simulink model "robust_controller"  (Simulink 7.2)
settings: Solver=FixedStepDiscrete  SolverMode=SingleTasking  StartTime=0  StopTime=inf  FixedStep=TS  RelTol=1e-3
PreLoadFcn:
  | param_nxtway_gs
values from neighbouring files (symbols this model uses):
  C_hh = [1 0]    [olp_robot_2dof.m]
undefined symbols (not defined in the file or in its folder): a_b, a_d, a_gc, a_gd, A_h, a_r, B_h, C_h, D_h, dst_thr, gp_max, k_phidot, k_sync, k_thetadot, log_count, pwm_gain, sound_dur, sound_freq, time_auto, time_start, ts1, ts2, ts3, turn_angle
libraries: ecrobot_nxt_lib x30, simulink x2
(part 1 of 2)
settings Model: Creator=y_yama  LastModifiedBy=Petko Petkov
settings DataIOCC: SaveOutput=off  SignalLogging=off  SaveTime=off
settings OptimizationCC: InlineParams=on  InlineInvariantSignals=on  EnforceIntegerDowncast=off  RollThreshold=2  StateBitsets=on  DataBitsets=on  UseTempVars=on  ZeroExternalMemoryAtStartup=off  ZeroInternalMemoryAtStartup=off  InitFltsAndDblsToZero=on  NoFixptDivByZeroProtection=on  EfficientFloat2IntCast=on  OptimizeModelRefInitCode=on  LifeSpan=1
settings DebuggingCC: ConsistencyChecking=warning  SignalInfNanChecking=warning  ReadBeforeWriteMsg=DisableAll  WriteAfterWriteMsg=DisableAll  WriteAfterReadMsg=DisableAll  AlgebraicLoopMsg=error  CheckExecutionContextPreStartOutputMsg=on  CheckExecutionContextRuntimeOutputMsg=on  SolverPrmCheckMsg=none  MultiTaskDSMMsg=warning  SingleTaskRateTransMsg=warning  TasksWithSamePriorityMsg=none  IntegerOverflowMsg=none  ParameterPrecisionLossMsg=none  UnconnectedInputMsg=error  UnconnectedOutputMsg=error  UnconnectedLineMsg=error  UniqueDataStoreMsg=error  BusObjectLabelMismatch=error  RootOutportRequireBusObject=error
settings HardwareCC: ProdIntDivRoundTo=Zero  ProdEndianess=LittleEndian  ProdHWDeviceType=ARM7  TargetHWDeviceType=32-bit Generic
settings ModelReferenceCC: ModelReferenceNumInstancesAllowed=Single
settings RTWCC: SystemTargetFile=ert.tlc  GenCodeOnly=on  GenerateMakefile=off  TemplateMakefile=ert_default_tmf  Description=Real-Time Workshop Embedded Coder (no auto configuration)  GenerateReport=on  RTWVerbose=off  ProcessScript=ert_make_rtw_hook  IncludeHyperlinkInReport=on  LaunchReport=on
settings CodeAppCC: ForceParamTrailComments=on  IgnoreCustomStorageClasses=off  MaxIdLength=63  SFDataObjDesc=on  CustomSymbolStrGlobalVar=rt$N$M  CustomSymbolStrType=$N$M  CustomSymbolStrFcn=$N$M$F  CustomSymbolStrMacro=$N$M  InsertBlockDesc=on
settings ERTTargetCC: TargetFcnLib=ansi_tfl_tmw.mat  TargetFunctionLibrary=GNU  MultiwordLength=2048  IncludeMdlTerminateFcn=off  SuppressErrorStatus=on  SupportAbsoluteTime=off  SupportNonFinite=off  SupportComplex=off  InlinedParameterPlacement=NonHierarchical  RootIOFormat=Structure reference  ERTCustomFileTemplate=example_file_process.tlc

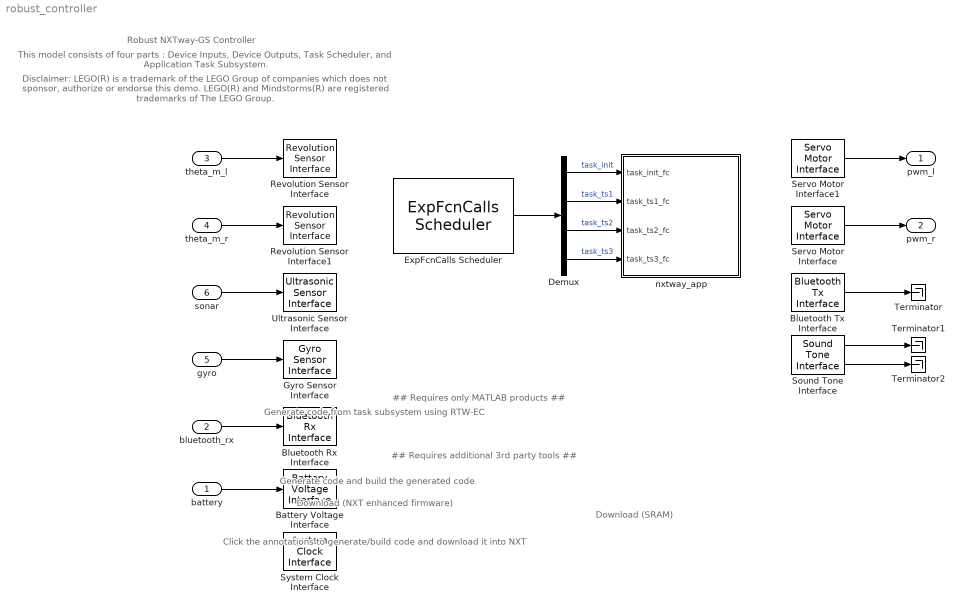
== system robust_controller ==
  note: Disclaimer:
      | LEGO(R) is a trademark of the LEGO Group of companies which does not sponsor, authorize or endorse this demo.
      | LEGO(R) and Mindstorms(R) are registered trademarks of The LEGO Group.
  note: Robust NXTway-GS Controller
  note: This model consists of four parts : Device Inputs, Device Outputs, Task Scheduler, and Application Task Subsystem.
  note: Generate code from task subsystem using RTW-EC
  note: Generate code and build the generated code
  note: ## Requires only MATLAB products ##
  note: ## Requires additional 3rd party tools ##
  note: Download (SRAM)
  note: Download (NXT enhanced firmware)
  note: Click the annotations to generate/build code and download it into NXT
  battery : Inport  DataType=uint16  OutDataType=sfix(16)  OutScaling=2^0  OutDataTypeStr=uint16
  bluetooth_rx : Inport  Port=2  DataType=uint8  OutDataType=sfix(16)  OutScaling=2^0  OutDataTypeStr=uint8
  theta_m_l : Inport  Port=3  DataType=int32  OutDataType=sfix(16)  OutScaling=2^0  OutDataTypeStr=int32
  theta_m_r : Inport  Port=4  DataType=int32  OutDataType=sfix(16)  OutScaling=2^0  OutDataTypeStr=int32
  gyro : Inport  Port=5  DataType=uint16  OutDataType=sfix(16)  OutScaling=2^0  OutDataTypeStr=uint16
  sonar : Inport  Port=6  DataType=int32  OutDataType=sfix(16)  OutScaling=2^0  OutDataTypeStr=int32
  Battery Voltage Interface : ecrobot_nxt_lib/Battery Voltage Interface  Priority=-1  SystemSampleTime=-1
      settings: AttributesFormatString=Priority = %<Priority>
  Bluetooth Rx Interface : ecrobot_nxt_lib/Bluetooth Rx Interface  Priority=-1  SystemSampleTime=-1
      settings: AttributesFormatString=Priority = %<Priority>
  Bluetooth Tx Interface : ecrobot_nxt_lib/Bluetooth Tx Interface  Priority=1  SystemSampleTime=-1
      settings: AttributesFormatString=Priority = %<Priority>
  Demux : Demux
  ExpFcnCalls Scheduler : ecrobot_nxt_lib/ExpFcnCalls Scheduler  Priority=0  fcname='task_init', 'task_ts1', 'task_ts2', 'task_ts3'  fctrigger=[0, ts1*1000, ts2*1000, ts3*1000]  ts=0.001  platform=OSEK  stacksize=[512, 512, 512, 512]  bd_mode=Slave
      settings: AttributesFormatString=Priority = %<Priority>
  Gyro Sensor Interface : ecrobot_nxt_lib/Gyro Sensor Interface  Priority=-1  SystemSampleTime=-1  ip=S4
      settings: AttributesFormatString=Port = %<ip>\nPriority = %<Priority>
  Revolution Sensor Interface : ecrobot_nxt_lib/Revolution Sensor Interface  Priority=-1  SystemSampleTime=-1  ip=C
      settings: AttributesFormatString=Port = %<ip>\nPriority = %<Priority>
  Revolution Sensor Interface1 : ecrobot_nxt_lib/Revolution Sensor Interface  Priority=-1  SystemSampleTime=-1  ip=B
      settings: AttributesFormatString=Port = %<ip>\nPriority = %<Priority>
  Servo Motor Interface : ecrobot_nxt_lib/Servo Motor Interface  Priority=1  SystemSampleTime=-1  ip=B  mode=Brake
      settings: AttributesFormatString=Port = %<ip>\nPriority = %<Priority>
  Servo Motor Interface1 : ecrobot_nxt_lib/Servo Motor Interface  Priority=1  SystemSampleTime=-1  ip=C  mode=Brake
      settings: AttributesFormatString=Port = %<ip>\nPriority = %<Priority>
  Sound Tone Interface : ecrobot_nxt_lib/Sound Tone  Interface  Priority=1  SystemSampleTime=-1
      settings: AttributesFormatString=Priority = %<Priority>
  System Clock Interface : ecrobot_nxt_lib/System Clock Interface  Priority=-1  SystemSampleTime=-1
      settings: AttributesFormatString=Priority = %<Priority>
  Terminator : Terminator
  Terminator1 : Terminator
  Terminator2 : Terminator
  Ultrasonic Sensor Interface : ecrobot_nxt_lib/Ultrasonic Sensor Interface  Priority=-1  SystemSampleTime=-1  ip=S2
      settings: AttributesFormatString=Port = %<ip>\nPriority = %<Priority>
  nxtway_app : Subsystem
  pwm_l : Outport  OutDataType=sfix(16)  OutScaling=2^0
  pwm_r : Outport  Port=2  OutDataType=sfix(16)  OutScaling=2^0
  wires:
  sonar/1 -> Ultrasonic Sensor Interface/1
  gyro/1 -> Gyro Sensor Interface/1
  theta_m_r/1 -> Revolution Sensor Interface1/1
  theta_m_l/1 -> Revolution Sensor Interface/1
  ExpFcnCalls Scheduler/1 -> Demux/1
  Bluetooth Tx Interface/1 -> Terminator/1
  Servo Motor Interface/1 -> pwm_r/1
  Servo Motor Interface1/1 -> pwm_l/1
  bluetooth_rx/1 -> Bluetooth Rx Interface/1
  battery/1 -> Battery Voltage Interface/1
  Demux/1 -> nxtway_app/1(task_init_fc)  "task_init"
  Demux/2 -> nxtway_app/2(task_ts1_fc)  "task_ts1"
  Demux/3 -> nxtway_app/3(task_ts2_fc)  "task_ts2"
  Demux/4 -> nxtway_app/4(task_ts3_fc)  "task_ts3"
  Sound Tone Interface/1 -> Terminator1/1
  Sound Tone Interface/2 -> Terminator2/1

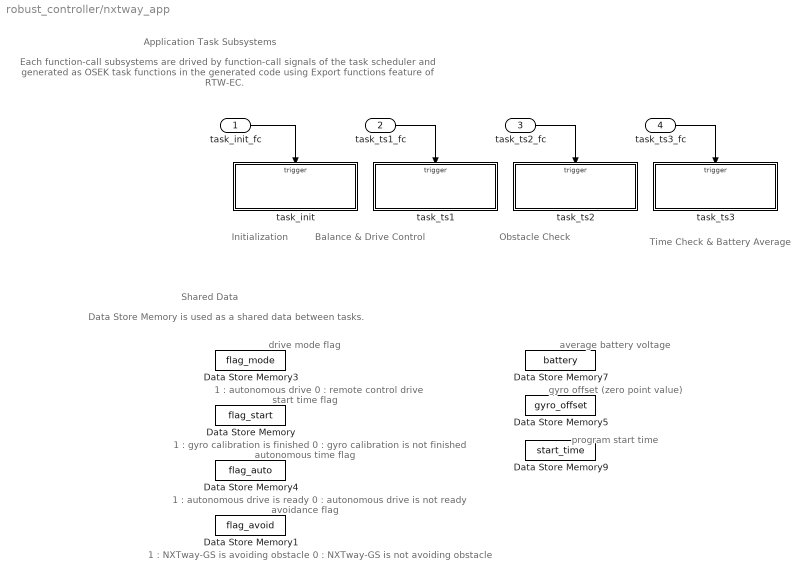
== system robust_controller/nxtway_app ==
  note: Application Task Subsystems
  note: Each function-call subsystems are drived by function-call signals of the task scheduler and
      | generated as OSEK task functions in the generated code using Export functions feature of RTW-EC.
  note: Initialization
  note: Balance & Drive Control
  note: Time Check &
      | Battery Average
  note: Shared Data
  note: Data Store Memory is used as a shared data between tasks.
  note: drive mode flag
  note: 1 : autonomous drive
      | 0 : remote control drive
  note: start time flag
  note: 1 : gyro calibration is finished
      | 0 : gyro calibration is not finished
  note: autonomous time flag
  note: 1 : autonomous drive is ready
      | 0 : autonomous drive is not ready
  note: average battery voltage
  note: gyro offset (zero point value)
  note: program start time
  note: Obstacle Check
  note: avoidance flag
  note: 1 : NXTway-GS is avoiding obstacle
      | 0 : NXTway-GS is not avoiding obstacle
  task_init_fc : Inport  OutDataType=sfix(16)  OutScaling=2^0
  task_ts1_fc : Inport  Port=2  OutDataType=sfix(16)  OutScaling=2^0
  task_ts2_fc : Inport  Port=3  OutDataType=sfix(16)  OutScaling=2^0
  task_ts3_fc : Inport  Port=4  OutDataType=sfix(16)  OutScaling=2^0
  Data Store Memory : DataStoreMemory  DataStoreName=flag_start  ReadBeforeWriteMsg=warning  WriteAfterWriteMsg=warning  WriteAfterReadMsg=warning  DataType=boolean  OutDataType=sfix(16)  OutScaling=2^0  OutDataTypeStr=boolean
      settings: AttributesFormatString=DataType = %<OutDataTypeStr>
  Data Store Memory1 : DataStoreMemory  DataStoreName=flag_avoid  ReadBeforeWriteMsg=warning  WriteAfterWriteMsg=warning  WriteAfterReadMsg=warning  DataType=boolean  OutDataType=sfix(16)  OutScaling=2^0  OutDataTypeStr=boolean
      settings: AttributesFormatString=DataType = %<OutDataTypeStr>
  Data Store Memory3 : DataStoreMemory  DataStoreName=flag_mode  ReadBeforeWriteMsg=warning  WriteAfterWriteMsg=warning  WriteAfterReadMsg=warning  DataType=boolean  OutDataType=sfix(16)  OutScaling=2^0  OutDataTypeStr=boolean
      settings: AttributesFormatString=DataType = %<OutDataTypeStr>
  Data Store Memory4 : DataStoreMemory  DataStoreName=flag_auto  ReadBeforeWriteMsg=warning  WriteAfterWriteMsg=warning  WriteAfterReadMsg=warning  DataType=boolean  OutDataType=sfix(16)  OutScaling=2^0  OutDataTypeStr=boolean
      settings: AttributesFormatString=DataType = %<OutDataTypeStr>
  Data Store Memory5 : DataStoreMemory  DataStoreName=gyro_offset  ReadBeforeWriteMsg=warning  WriteAfterWriteMsg=warning  WriteAfterReadMsg=warning  DataType=single  OutDataType=sfix(16)  OutScaling=2^0  OutDataTypeStr=single
      settings: AttributesFormatString=DataType = %<OutDataTypeStr>
  Data Store Memory7 : DataStoreMemory  DataStoreName=battery  ReadBeforeWriteMsg=warning  WriteAfterWriteMsg=warning  WriteAfterReadMsg=warning  DataType=single  OutDataType=sfix(16)  OutScaling=2^0  OutDataTypeStr=single
      settings: AttributesFormatString=DataType = %<OutDataTypeStr>
  Data Store Memory9 : DataStoreMemory  DataStoreName=start_time  ReadBeforeWriteMsg=warning  WriteAfterWriteMsg=warning  WriteAfterReadMsg=warning  DataType=uint32  OutDataType=sfix(16)  OutScaling=2^0  OutDataTypeStr=uint32
      settings: AttributesFormatString=DataType = %<OutDataTypeStr>
  task_init : Subsystem  TreatAsAtomicUnit=on
  task_ts1 : Subsystem  TreatAsAtomicUnit=on
  task_ts2 : Subsystem  TreatAsAtomicUnit=on
  task_ts3 : Subsystem  TreatAsAtomicUnit=on
  wires:
  task_init_fc/1 -> task_init/Trigger
  task_ts1_fc/1 -> task_ts1/Trigger
  task_ts3_fc/1 -> task_ts3/Trigger
  task_ts2_fc/1 -> task_ts2/Trigger

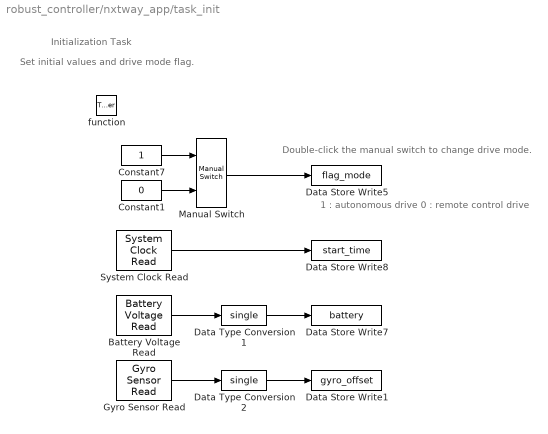
== system robust_controller/nxtway_app/task_init ==
  note: Initialization Task
  note: Set initial values and drive mode flag.
  note: Double-click the manual switch
      |  to change drive mode.
  note: 1 : autonomous drive
      | 0 : remote control drive
  function : TriggerPort  TriggerType=function-call
  Battery Voltage Read : ecrobot_nxt_lib/Battery Voltage Read  SystemSampleTime=-1
  Constant1 : Constant  Value=0  OutDataTypeMode=boolean  OutDataType=sfix(16)  OutScaling=2^0  OutDataTypeStr=boolean  SampleTime=-1
      settings: AttributesFormatString=DataType = %<OutDataTypeStr>
  Constant7 : Constant  OutDataTypeMode=boolean  OutDataType=sfix(16)  OutScaling=2^0  OutDataTypeStr=boolean  SampleTime=-1
      settings: AttributesFormatString=DataType = %<OutDataTypeStr>
  Data Store Write1 : DataStoreWrite  DataStoreName=gyro_offset  SampleTime=-1
  Data Store Write5 : DataStoreWrite  DataStoreName=flag_mode  SampleTime=-1
  Data Store Write7 : DataStoreWrite  DataStoreName=battery  SampleTime=-1
  Data Store Write8 : DataStoreWrite  DataStoreName=start_time  SampleTime=-1
  Data Type Conversion1 : DataTypeConversion  OutDataTypeMode=single  OutDataType=sfix(16)  OutScaling=2^0  OutDataTypeStr=single  RndMeth=Simplest
      settings: AttributesFormatString=Round = %<RndMeth>
  Data Type Conversion2 : DataTypeConversion  OutDataTypeMode=single  OutDataType=sfix(16)  OutScaling=2^0  OutDataTypeStr=single  RndMeth=Simplest
      settings: AttributesFormatString=Round = %<RndMeth>
  Gyro Sensor Read : ecrobot_nxt_lib/Gyro Sensor Read  SystemSampleTime=-1  ip=S4
      settings: AttributesFormatString=Port = %<ip>
  Manual Switch : simulink/Signal Routing/Manual Switch  SystemSampleTime=-1  sw=0  action=0  varsize=off
  System Clock Read : ecrobot_nxt_lib/System Clock Read  SystemSampleTime=-1
  wires:
  Gyro Sensor Read/1 -> Data Type Conversion2/1
  Data Type Conversion2/1 -> Data Store Write1/1
  Battery Voltage Read/1 -> Data Type Conversion1/1
  Data Type Conversion1/1 -> Data Store Write7/1
  Constant7/1 -> Manual Switch/1
  Constant1/1 -> Manual Switch/2
  Manual Switch/1 -> Data Store Write5/1
  System Clock Read/1 -> Data Store Write8/1

== system robust_controller/nxtway_app/task_ts1 ==
  note: Balance & Drive Control Task
  note: Control NXTway-GS to balance itself and drive autonomously or
      | by remote control after gyro calibration.
  function : TriggerPort  TriggerType=function-call
  Balance & Drive Control : Subsystem
  Data Store Read : DataStoreRead  DataStoreName=flag_start  SampleTime=-1
  Gyro Calibration : Subsystem  TreatAsAtomicUnit=on
  Logical Operator : Logic  Operator=NOT  AllPortsSameDT=off  OutDataTypeMode=boolean  OutDataTypeStr=boolean
  wires:
  Data Store Read/1 -> Logical Operator/1, Balance & Drive Control/Enable
  Logical Operator/1 -> Gyro Calibration/Enable

== system robust_controller/nxtway_app/task_ts2 ==
  note: Get the distance between NXTway-GS and obstacle using the ultrasonic sensor.
      | NXTway-GS rotates right in autonomous drive mode and runs backward in remote
      | control drive mode when the distance is under the threshold.
  note: Obstacle Check Task
  function : TriggerPort  TriggerType=function-call
  Autonomous Drive : Subsystem
  Data Store Read1 : DataStoreRead  DataStoreName=flag_mode  SampleTime=-1
  Logical Operator : Logic  Operator=NOT  AllPortsSameDT=off  OutDataTypeMode=boolean  OutDataTypeStr=boolean
  Remote Control Drive : Subsystem
  wires:
  Logical Operator/1 -> Remote Control Drive/Enable
  Data Store Read1/1 -> Logical Operator/1, Autonomous Drive/Enable

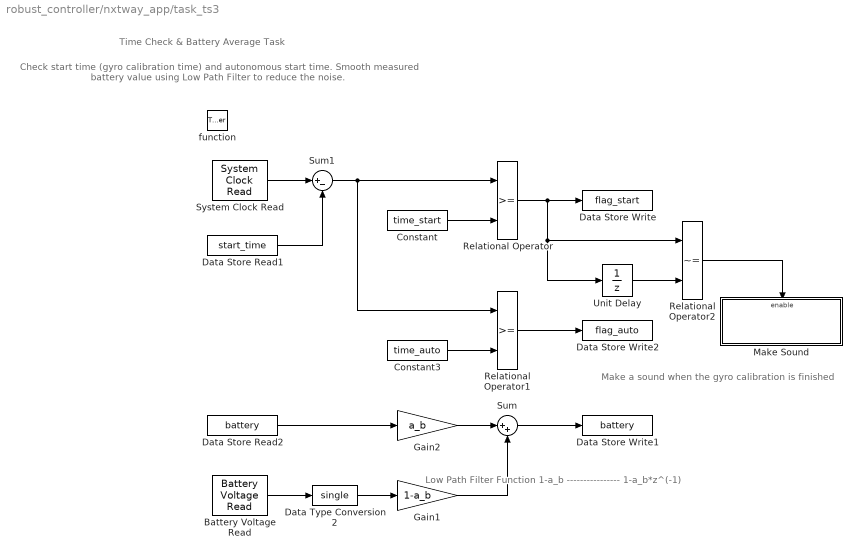
== system robust_controller/nxtway_app/task_ts3 ==
  note: Time Check & Battery Average Task
  note: Check start time (gyro calibration time) and autonomous start time.
      | Smooth measured battery value using Low Path Filter to reduce the noise.
  note: Low Path Filter Function
      |               1-a_b
      |          ----------------
      |          1-a_b*z^(-1)
  note: Make a sound when the
      | gyro calibration is finished
  function : TriggerPort  TriggerType=function-call
  Battery Voltage Read : ecrobot_nxt_lib/Battery Voltage Read  SystemSampleTime=-1
  Constant : Constant  Value=time_start  OutDataTypeMode=uint32  OutDataType=sfix(16)  OutScaling=2^0  OutDataTypeStr=uint32  SampleTime=-1
      settings: AttributesFormatString=DataType = %<OutDataTypeStr>
  Constant3 : Constant  Value=time_auto  OutDataTypeMode=uint32  OutDataType=sfix(16)  OutScaling=2^0  OutDataTypeStr=uint32  SampleTime=-1
      settings: AttributesFormatString=DataType = %<OutDataTypeStr>
  Data Store Read1 : DataStoreRead  DataStoreName=start_time  SampleTime=-1
  Data Store Read2 : DataStoreRead  DataStoreName=battery  SampleTime=-1
  Data Store Write : DataStoreWrite  DataStoreName=flag_start  SampleTime=-1
  Data Store Write1 : DataStoreWrite  DataStoreName=battery  SampleTime=-1
  Data Store Write2 : DataStoreWrite  DataStoreName=flag_auto  SampleTime=-1
  Data Type Conversion2 : DataTypeConversion  OutDataTypeMode=single  OutDataType=sfix(16)  OutScaling=2^0  OutDataTypeStr=single  RndMeth=Simplest
      settings: AttributesFormatString=Round = %<RndMeth>
  Gain1 : Gain  Gain=1-a_b  ParameterDataType=sfix(16)  ParameterScaling=2^0  OutDataType=sfix(16)  OutScaling=2^0  OutDataTypeStr=Inherit: Same as input  ParamDataTypeStr=Inherit: Same as input
  Gain2 : Gain  Gain=a_b  ParameterDataType=sfix(16)  ParameterScaling=2^0  OutDataType=sfix(16)  OutScaling=2^0  OutDataTypeStr=Inherit: Same as input  ParamDataTypeStr=Inherit: Same as input
  Make Sound : Subsystem
  Relational Operator : RelationalOperator  LogicOutDataTypeMode=boolean  OutDataTypeStr=boolean
  Relational Operator1 : RelationalOperator  LogicOutDataTypeMode=boolean  OutDataTypeStr=boolean
  Relational Operator2 : RelationalOperator  Operator=~=  LogicOutDataTypeMode=boolean  OutDataTypeStr=boolean
  Sum : Sum  Inputs=|++  OutDataType=sfix(16)  OutScaling=2^0  OutDataTypeStr=Inherit: Same as first input
  Sum1 : Sum  Inputs=|+-  OutDataType=sfix(16)  OutScaling=2^0  OutDataTypeStr=Inherit: Same as first input
  System Clock Read : ecrobot_nxt_lib/System Clock Read  SystemSampleTime=-1
  Unit Delay : UnitDelay  SampleTime=-1
  wires:
  Data Type Conversion2/1 -> Gain1/1
  Sum/1 -> Data Store Write1/1
  Data Store Read2/1 -> Gain2/1
  Gain2/1 -> Sum/1
  Gain1/1 -> Sum/2
  Battery Voltage Read/1 -> Data Type Conversion2/1
  Constant/1 -> Relational Operator/2
  Relational Operator/1 -> Data Store Write/1, Unit Delay/1, Relational Operator2/1
  Relational Operator1/1 -> Data Store Write2/1
  Constant3/1 -> Relational Operator1/2
  System Clock Read/1 -> Sum1/1
  Sum1/1 -> Relational Operator/1, Relational Operator1/1
  Data Store Read1/1 -> Sum1/2
  Unit Delay/1 -> Relational Operator2/2
  Relational Operator2/1 -> Make Sound/Enable

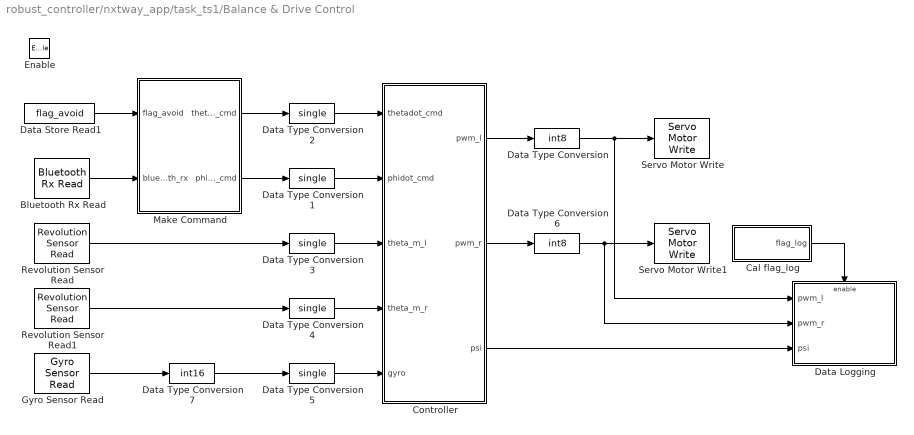
== system robust_controller/nxtway_app/task_ts1/Balance & Drive Control ==
  Enable : EnablePort
  Bluetooth Rx Read : ecrobot_nxt_lib/Bluetooth Rx Read
  Cal flag_log : Subsystem
  Controller : Subsystem
  Data Logging : Subsystem  TreatAsAtomicUnit=on
  Data Store Read1 : DataStoreRead  DataStoreName=flag_avoid  SampleTime=-1
  Data Type Conversion : DataTypeConversion  OutDataTypeMode=int8  OutDataType=sfix(16)  OutScaling=2^0  OutDataTypeStr=int8  RndMeth=Simplest
      settings: AttributesFormatString=Round = %<RndMeth>
  Data Type Conversion{1..5} (5 alike) : DataTypeConversion  OutDataTypeMode=single  OutDataType=sfix(16)  OutScaling=2^0  OutDataTypeStr=single  RndMeth=Simplest
      settings: AttributesFormatString=Round = %<RndMeth>
  Data Type Conversion6 : DataTypeConversion  OutDataTypeMode=int8  OutDataType=sfix(16)  OutScaling=2^0  OutDataTypeStr=int8  RndMeth=Simplest
      settings: AttributesFormatString=Round = %<RndMeth>
  Data Type Conversion7 : DataTypeConversion  OutDataTypeMode=int16  OutDataType=sfix(16)  OutScaling=2^0  OutDataTypeStr=int16  RndMeth=Simplest
      settings: AttributesFormatString=Round = %<RndMeth>
  Gyro Sensor Read : ecrobot_nxt_lib/Gyro Sensor Read  SystemSampleTime=-1  ip=S4
      settings: AttributesFormatString=Port = %<ip>
  Make Command : Subsystem
  Revolution Sensor Read : ecrobot_nxt_lib/Revolution Sensor Read  SystemSampleTime=-1  ip=C
      settings: AttributesFormatString=Port = %<ip>
  Revolution Sensor Read1 : ecrobot_nxt_lib/Revolution Sensor Read  SystemSampleTime=-1  ip=B
      settings: AttributesFormatString=Port = %<ip>
  Servo Motor Write : ecrobot_nxt_lib/Servo Motor Write  SystemSampleTime=-1  ip=C
      settings: AttributesFormatString=Port = %<ip>
  Servo Motor Write1 : ecrobot_nxt_lib/Servo Motor Write  SystemSampleTime=-1  ip=B
      settings: AttributesFormatString=Port = %<ip>
  wires:
  Controller/1(pwm_l) -> Data Type Conversion/1
  Controller/2(pwm_r) -> Data Type Conversion6/1
  Make Command/1(thetadot_cmd) -> Data Type Conversion2/1
  Make Command/2(phidot_cmd) -> Data Type Conversion1/1
  Revolution Sensor Read1/1 -> Data Type Conversion4/1
  Revolution Sensor Read/1 -> Data Type Conversion3/1
  Bluetooth Rx Read/1 -> Make Command/2(bluetooth_rx)
  Data Type Conversion3/1 -> Controller/3(theta_m_l)
  Data Type Conversion4/1 -> Controller/4(theta_m_r)
  Data Type Conversion5/1 -> Controller/5(gyro)
  Data Type Conversion/1 -> Servo Motor Write/1, Data Logging/1(pwm_l)
  Data Type Conversion6/1 -> Servo Motor Write1/1, Data Logging/2(pwm_r)
  Cal flag_log/1(flag_log) -> Data Logging/Enable
  Controller/3(psi) -> Data Logging/3(psi)
  Data Type Conversion1/1 -> Controller/2(phidot_cmd)
  Data Type Conversion2/1 -> Controller/1(thetadot_cmd)
  Data Store Read1/1 -> Make Command/1(flag_avoid)
  Gyro Sensor Read/1 -> Data Type Conversion7/1
  Data Type Conversion7/1 -> Data Type Conversion5/1

== system robust_controller/nxtway_app/task_ts1/Gyro Calibration ==
  note: Low Path Filter Function
      |               1-a_gc
      |          ----------------
      |          1-a_gc*z^(-1)
  note: Calculate gyro offset (zero point value).
  Enable : EnablePort
  Data Store Read2 : DataStoreRead  DataStoreName=gyro_offset  SampleTime=-1
  Data Store Write1 : DataStoreWrite  DataStoreName=gyro_offset  SampleTime=-1
  Data Type Conversion2 : DataTypeConversion  OutDataTypeMode=single  OutDataType=sfix(16)  OutScaling=2^0  OutDataTypeStr=single  RndMeth=Simplest
      settings: AttributesFormatString=Round = %<RndMeth>
  Gain1 : Gain  Gain=1-a_gc  ParameterDataType=sfix(16)  ParameterScaling=2^0  OutDataType=sfix(16)  OutScaling=2^0  OutDataTypeStr=Inherit: Same as input  ParamDataTypeStr=Inherit: Same as input
  Gain4 : Gain  Gain=a_gc  ParameterDataType=sfix(16)  ParameterScaling=2^0  OutDataType=sfix(16)  OutScaling=2^0  OutDataTypeStr=Inherit: Same as input  ParamDataTypeStr=Inherit: Same as input
  Gyro Sensor Read : ecrobot_nxt_lib/Gyro Sensor Read  SystemSampleTime=-1  ip=S4
      settings: AttributesFormatString=Port = %<ip>
  Sum : Sum  Inputs=|++  OutDataType=sfix(16)  OutScaling=2^0  OutDataTypeStr=Inherit: Same as first input
  wires:
  Gyro Sensor Read/1 -> Data Type Conversion2/1
  Data Type Conversion2/1 -> Gain1/1
  Sum/1 -> Data Store Write1/1
  Data Store Read2/1 -> Gain4/1
  Gain4/1 -> Sum/1
  Gain1/1 -> Sum/2

== system robust_controller/nxtway_app/task_ts2/Autonomous Drive ==
  Enable : EnablePort
  Data Store Read2 : DataStoreRead  DataStoreName=flag_avoid  SampleTime=-1
  Forward Run : Subsystem
  Logical Operator1 : Logic  Operator=NOT  AllPortsSameDT=off  OutDataTypeMode=boolean  OutDataTypeStr=boolean
  Rotate Right : Subsystem
  wires:
  Forward Run/1(theta_m_l) -> Rotate Right/1(theta_m_l)
  Logical Operator1/1 -> Forward Run/Enable
  Data Store Read2/1 -> Logical Operator1/1, Rotate Right/Enable

== system robust_controller/nxtway_app/task_ts2/Remote Control Drive ==
  Enable : EnablePort
  Constant : Constant  Value=dst_thr  OutDataTypeMode=int32  OutDataType=sfix(16)  OutScaling=2^0  OutDataTypeStr=int32  SampleTime=-1
      settings: AttributesFormatString=DataType = %<OutDataTypeStr>
  Data Store Write1 : DataStoreWrite  DataStoreName=flag_avoid  SampleTime=-1
  Relational Operator : RelationalOperator  Operator=<=  LogicOutDataTypeMode=boolean  OutDataTypeStr=boolean
  Ultrasonic Sensor Read : ecrobot_nxt_lib/Ultrasonic Sensor Read  SystemSampleTime=-1  ip=S2
      settings: AttributesFormatString=Port = %<ip>
  wires:
  Ultrasonic Sensor Read/1 -> Relational Operator/1
  Relational Operator/1 -> Data Store Write1/1
  Constant/1 -> Relational Operator/2

== system robust_controller/nxtway_app/task_ts3/Make Sound ==
  Enable : EnablePort
  Constant : Constant  Value=sound_freq  OutDataTypeMode=uint32  OutDataType=sfix(16)  OutScaling=2^0  OutDataTypeStr=uint32  SampleTime=-1
      settings: AttributesFormatString=DataType = %<OutDataTypeStr>
  Constant1 : Constant  Value=sound_dur  OutDataTypeMode=uint32  OutDataType=sfix(16)  OutScaling=2^0  OutDataTypeStr=uint32  SampleTime=-1
      settings: AttributesFormatString=DataType = %<OutDataTypeStr>
  Sound Tone Write : ecrobot_nxt_lib/Sound Tone Write
  wires:
  Constant/1 -> Sound Tone Write/1
  Constant1/1 -> Sound Tone Write/2

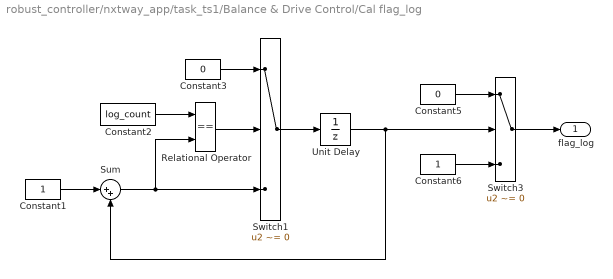
== system robust_controller/nxtway_app/task_ts1/Balance & Drive Control/Cal flag_log ==
  Constant1 : Constant  VectorParams1D=off  OutDataTypeMode=uint8  OutDataType=FIXDT  OutScaling=2^0  OutDataTypeStr=uint8  SampleTime=-1
      settings: AttributesFormatString=DataType = %<OutDataTypeStr>
  Constant2 : Constant  Value=log_count  VectorParams1D=off  OutDataTypeMode=uint8  OutDataType=FIXDT  OutScaling=2^0  OutDataTypeStr=uint8  SampleTime=-1
      settings: AttributesFormatString=DataType = %<OutDataTypeStr>
  Constant3 : Constant  Value=0  VectorParams1D=off  OutDataTypeMode=uint8  OutDataType=FIXDT  OutScaling=2^0  OutDataTypeStr=uint8  SampleTime=-1
      settings: AttributesFormatString=DataType = %<OutDataTypeStr>
  Constant5 : Constant  Value=0  OutDataTypeMode=boolean  OutDataType=sfix(16)  OutScaling=2^0  OutDataTypeStr=boolean  SampleTime=-1
      settings: AttributesFormatString=DataType = %<OutDataTypeStr>
  Constant6 : Constant  OutDataTypeMode=boolean  OutDataType=sfix(16)  OutScaling=2^0  OutDataTypeStr=boolean  SampleTime=-1
      settings: AttributesFormatString=DataType = %<OutDataTypeStr>
  Relational Operator : RelationalOperator  Operator===  LogicOutDataTypeMode=boolean  OutDataTypeStr=boolean
  Sum : Sum  Inputs=|++  OutDataType=sfix(16)  OutScaling=2^0  OutDataTypeStr=Inherit: Same as first input
  Switch1 : Switch  Criteria=u2 ~= 0  OutDataType=sfix(16)  OutScaling=2^0
  Switch3 : Switch  Criteria=u2 ~= 0  OutDataType=sfix(16)  OutScaling=2^0
  Unit Delay : UnitDelay  SampleTime=-1
  flag_log : Outport
  wires:
  Switch3/1 -> flag_log/1
  Constant5/1 -> Switch3/1
  Constant6/1 -> Switch3/3
  Switch1/1 -> Unit Delay/1
  Unit Delay/1 -> Sum/2, Switch3/2
  Constant1/1 -> Sum/1
  Constant3/1 -> Switch1/1
  Sum/1 -> Switch1/3, Relational Operator/2
  Constant2/1 -> Relational Operator/1
  Relational Operator/1 -> Switch1/2

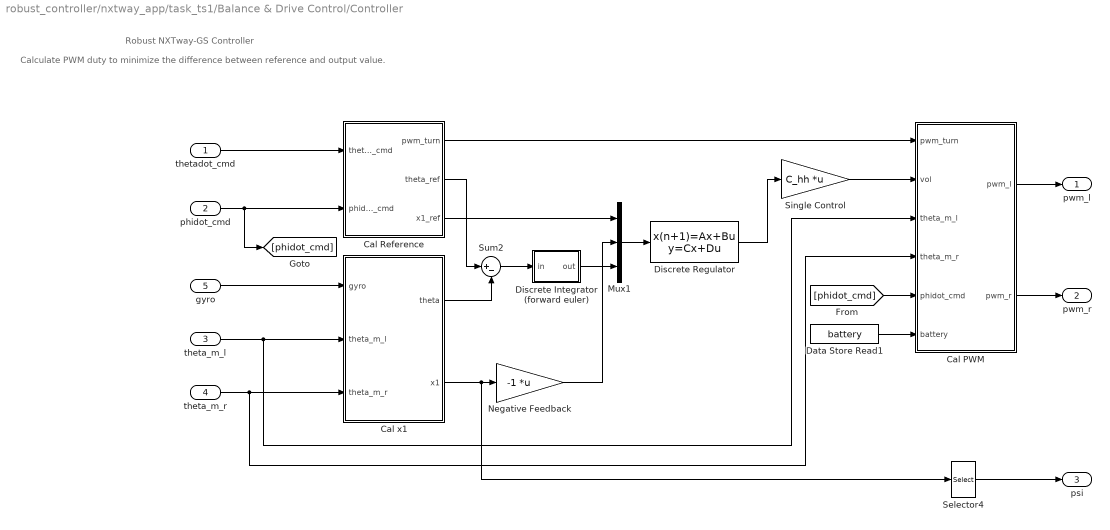
== system robust_controller/nxtway_app/task_ts1/Balance & Drive Control/Controller ==
  note: Robust NXTway-GS Controller
  note: Calculate PWM duty to minimize the difference between reference and output value.
  thetadot_cmd : Inport
  phidot_cmd : Inport  Port=2
  theta_m_l : Inport  Port=3
  theta_m_r : Inport  Port=4
  gyro : Inport  Port=5
  Cal PWM : Subsystem
  Cal Reference : Subsystem
  Cal x1 : Subsystem
  Data Store Read1 : DataStoreRead  DataStoreName=battery  SampleTime=-1
  Discrete Integrator (forward euler) : Subsystem
  "Discrete Regulator " : DiscreteStateSpace  A=A_h  B=B_h  C=C_h  D=D_h  SampleTime=-1
  Mux1 : Mux  Inputs=3
  Negative Feedback : Gain  Gain=-1  Multiplication=Matrix(K*u)  ParameterDataType=sfix(16)  ParameterScaling=2^0  OutDataType=sfix(16)  OutScaling=2^0  OutDataTypeStr=Inherit: Same as input  ParamDataTypeStr=Inherit: Same as input
  Selector4 : Selector  InputPortWidth=4  IndexOptions=Index vector (dialog)  Indices=2  OutputSizes=1
  "Single Control " : Gain  Gain=C_hh  Multiplication=Matrix(K*u)  ParameterDataType=sfix(16)  ParameterScaling=2^0  OutDataType=sfix(16)  OutScaling=2^0  OutDataTypeStr=Inherit: Same as input  ParamDataTypeStr=Inherit: Same as input
  Sum2 : Sum  Inputs=|+-  OutDataType=sfix(16)  OutScaling=2^0  OutDataTypeStr=Inherit: Same as first input
  pwm_l : Outport
  pwm_r : Outport  Port=2
  psi : Outport  Port=3
  wires:
  gyro/1 -> Cal x1/1(gyro)
  theta_m_l/1 -> Cal PWM/3(theta_m_l), Cal x1/2(theta_m_l)
  Cal PWM/2(pwm_r) -> pwm_r/1
  Cal PWM/1(pwm_l) -> pwm_l/1
  Cal Reference/1(pwm_turn) -> Cal PWM/1(pwm_turn)
  thetadot_cmd/1 -> Cal Reference/1(thetadot_cmd)
  phidot_cmd/1 -> Cal Reference/2(phidot_cmd), [phidot_cmd]
  Data Store Read1/1 -> Cal PWM/6(battery)
  theta_m_r/1 -> Cal x1/3(theta_m_r), Cal PWM/4(theta_m_r)
  Cal x1/2(x1) -> Negative Feedback/1, Selector4/1
  Selector4/1 -> psi/1
  [phidot_cmd] -> Cal PWM/5(phidot_cmd)
  Mux1/1 -> "Discrete Regulator "/1
  Cal x1/1(theta) -> Sum2/2
  Cal Reference/2(theta_ref) -> Sum2/1
  "Single Control "/1 -> Cal PWM/2(vol)
  "Discrete Regulator "/1 -> "Single Control "/1
  Sum2/1 -> Discrete Integrator (forward euler)/1(in)
  Cal Reference/3(x1_ref) -> Mux1/1
  Negative Feedback/1 -> Mux1/2
  Discrete Integrator (forward euler)/1(out) -> Mux1/3

== system robust_controller/nxtway_app/task_ts1/Balance & Drive Control/Data Logging ==
  note: Data Logging
  note: Log the body angle using NXT GamePad ADC Data Logger.
  pwm_l : Inport  OutDataType=sfix(16)  OutScaling=2^0
  pwm_r : Inport  Port=2  OutDataType=sfix(16)  OutScaling=2^0
  psi : Inport  Port=3  OutDataType=sfix(16)  OutScaling=2^0
  Enable : EnablePort
  Data Type Conversion2 : DataTypeConversion  OutDataTypeMode=int16  OutDataType=sfix(16)  OutScaling=2^0  OutDataTypeStr=int16  RndMeth=Nearest
      settings: AttributesFormatString=Round = %<RndMeth>
  Ground1 : Ground
  NXT GamePad  ADC Data Logger : ecrobot_nxt_lib/NXT GamePad  ADC Data Logger
  Scaling : Subsystem
  wires:
  Scaling/1(psi_int) -> Data Type Conversion2/1
  Data Type Conversion2/1 -> NXT GamePad  ADC Data Logger/3
  psi/1 -> Scaling/1(psi_single)
  pwm_l/1 -> NXT GamePad  ADC Data Logger/1
  pwm_r/1 -> NXT GamePad  ADC Data Logger/2
  Ground1/1 -> NXT GamePad  ADC Data Logger/6, NXT GamePad  ADC Data Logger/4, NXT GamePad  ADC Data Logger/5

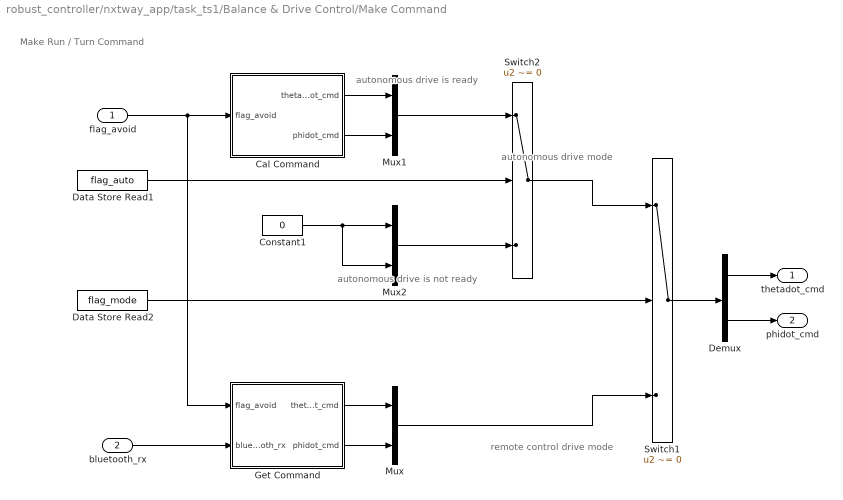
== system robust_controller/nxtway_app/task_ts1/Balance & Drive Control/Make Command ==
  note: Make Run / Turn Command
  note: autonomous
      | drive mode
  note: remote control
      | drive mode
  note: autonomous
      | drive is ready
  note: autonomous
      | drive is not ready
  flag_avoid : Inport
  bluetooth_rx : Inport  Port=2  OutDataType=sfix(16)  OutScaling=2^0
  Cal Command : Subsystem
  Constant1 : Constant  Value=0  VectorParams1D=off  OutDataTypeMode=int8  OutDataType=FIXDT  OutScaling=2^0  OutDataTypeStr=int8  SampleTime=-1
      settings: AttributesFormatString=DataType = %<OutDataTypeStr>
  Data Store Read1 : DataStoreRead  DataStoreName=flag_auto  SampleTime=-1
  Data Store Read2 : DataStoreRead  DataStoreName=flag_mode  SampleTime=-1
  Demux : Demux  Outputs=2
  Get Command : Subsystem
  Mux : Mux  Inputs=2
  Mux1 : Mux  Inputs=2
  Mux2 : Mux  Inputs=2
  Switch1 : Switch  Criteria=u2 ~= 0  OutDataType=sfix(16)  OutScaling=2^0
  Switch2 : Switch  Criteria=u2 ~= 0  OutDataType=sfix(16)  OutScaling=2^0
  thetadot_cmd : Outport  OutDataType=sfix(16)  OutScaling=2^0
  phidot_cmd : Outport  Port=2  OutDataType=sfix(16)  OutScaling=2^0
  wires:
  bluetooth_rx/1 -> Get Command/2(bluetooth_rx)
  Data Store Read2/1 -> Switch1/2
  Get Command/1(thetadot_cmd) -> Mux/1
  Get Command/2(phidot_cmd) -> Mux/2
  Demux/2 -> phidot_cmd/1
  Demux/1 -> thetadot_cmd/1
  Cal Command/1(thetadot_cmd) -> Mux1/1
  Cal Command/2(phidot_cmd) -> Mux1/2
  Mux/1 -> Switch1/3
  Data Store Read1/1 -> Switch2/2
  Mux1/1 -> Switch2/1
  Constant1/1 -> Mux2/1, Mux2/2
  Mux2/1 -> Switch2/3
  Switch2/1 -> Switch1/1
  flag_avoid/1 -> Cal Command/1(flag_avoid), Get Command/1(flag_avoid)
  Switch1/1 -> Demux/1

== system robust_controller/nxtway_app/task_ts2/Autonomous Drive/Forward Run ==
  note: Set flag_avoid and store left motor revolution angle.
  Enable : EnablePort
  Constant : Constant  Value=dst_thr  OutDataTypeMode=int32  OutDataType=sfix(16)  OutScaling=2^0  OutDataTypeStr=int32  SampleTime=-1
      settings: AttributesFormatString=DataType = %<OutDataTypeStr>
  Data Store Write1 : DataStoreWrite  DataStoreName=flag_avoid  SampleTime=-1
  Relational Operator : RelationalOperator  Operator=<=  LogicOutDataTypeMode=boolean  OutDataTypeStr=boolean
  Revolution Sensor Read : ecrobot_nxt_lib/Revolution Sensor Read  SystemSampleTime=-1  ip=C
      settings: AttributesFormatString=Port = %<ip>
  Ultrasonic Sensor Read : ecrobot_nxt_lib/Ultrasonic Sensor Read  SystemSampleTime=-1  ip=S2
      settings: AttributesFormatString=Port = %<ip>
  theta_m_l : Outport
  wires:
  Relational Operator/1 -> Data Store Write1/1
  Constant/1 -> Relational Operator/2
  Ultrasonic Sensor Read/1 -> Relational Operator/1
  Revolution Sensor Read/1 -> theta_m_l/1

== system robust_controller/nxtway_app/task_ts2/Autonomous Drive/Rotate Right ==
  note: NXTway-GS rotates right by turn_angle [deg].
  theta_m_l : Inport
  Enable : EnablePort
  Constant1 : Constant  Value=turn_angle  OutDataTypeMode=int32  OutDataType=sfix(16)  OutScaling=2^0  OutDataTypeStr=int32  SampleTime=-1
      settings: AttributesFormatString=DataType = %<OutDataTypeStr>
  Data Store Write1 : DataStoreWrite  DataStoreName=flag_avoid  SampleTime=-1
  Relational Operator1 : RelationalOperator  Operator=<=  LogicOutDataTypeMode=boolean  OutDataTypeStr=boolean
  Revolution Sensor Read : ecrobot_nxt_lib/Revolution Sensor Read  SystemSampleTime=-1  ip=C
      settings: AttributesFormatString=Port = %<ip>
  Sum1 : Sum  Inputs=|+-  OutDataType=sfix(16)  OutScaling=2^0  OutDataTypeStr=Inherit: Same as first input
  wires:
  Relational Operator1/1 -> Data Store Write1/1
  theta_m_l/1 -> Sum1/2
  Sum1/1 -> Relational Operator1/1
  Revolution Sensor Read/1 -> Sum1/1
  Constant1/1 -> Relational Operator1/2

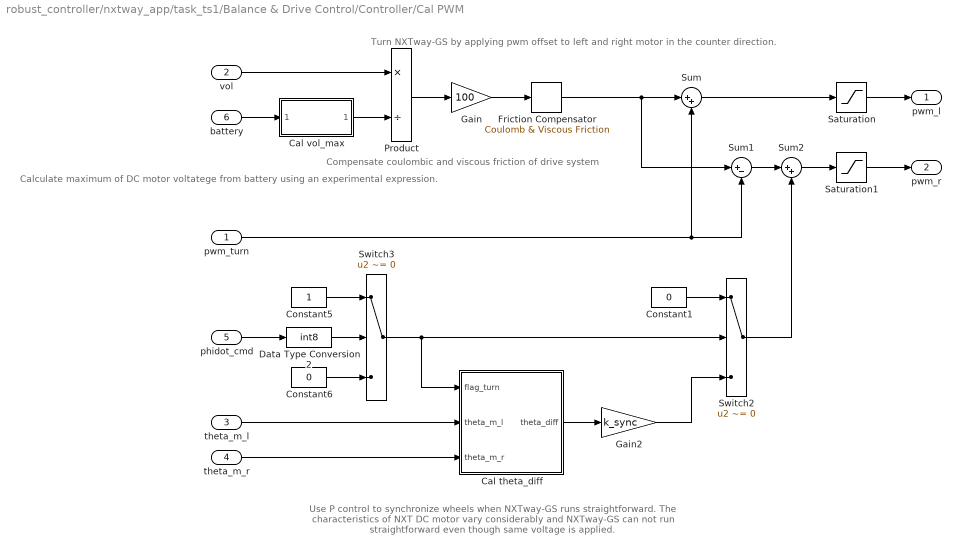
== system robust_controller/nxtway_app/task_ts1/Balance & Drive Control/Controller/Cal PWM ==
  note: Calculate maximum of DC motor
      | voltatege from battery using an
      | experimental expression.
  note: Use P control to synchronize wheels when NXTway-GS runs straightforward.
      | The characteristics of NXT DC motor vary considerably and NXTway-GS can not
      | run straightforward even though same voltage is applied.
  note: Turn NXTway-GS by applying pwm offset
      | to left and right motor in the counter direction.
  note: Compensate coulombic and
      | viscous friction of drive system
  pwm_turn : Inport
  vol : Inport  Port=2  OutDataType=sfix(16)  OutScaling=2^0
  theta_m_l : Inport  Port=3  OutDataType=sfix(16)  OutScaling=2^0
  theta_m_r : Inport  Port=4  OutDataType=sfix(16)  OutScaling=2^0
  phidot_cmd : Inport  Port=5
  battery : Inport  Port=6  OutDataType=sfix(16)  OutScaling=2^0
  Cal theta_diff : Subsystem
  Cal vol_max : Subsystem
  Constant1 : Constant  Value=0  OutDataTypeMode=single  OutDataType=sfix(16)  OutScaling=2^0  OutDataTypeStr=single  SampleTime=-1
      settings: AttributesFormatString=DataType = %<OutDataTypeStr>
  Constant5 : Constant  OutDataTypeMode=boolean  OutDataType=sfix(16)  OutScaling=2^0  OutDataTypeStr=boolean  SampleTime=-1
      settings: AttributesFormatString=DataType = %<OutDataTypeStr>
  Constant6 : Constant  Value=0  OutDataTypeMode=boolean  OutDataType=sfix(16)  OutScaling=2^0  OutDataTypeStr=boolean  SampleTime=-1
      settings: AttributesFormatString=DataType = %<OutDataTypeStr>
  Data Type Conversion2 : DataTypeConversion  OutDataTypeMode=int8  OutDataType=sfix(16)  OutScaling=2^0  OutDataTypeStr=int8  RndMeth=Simplest
      settings: AttributesFormatString=Round = %<RndMeth>
  Friction Compensator : simulink/Discontinuities/Coulomb & Viscous Friction  SystemSampleTime=-1  offset=pwm_offset  gain=pwm_gain
      settings: AttributesFormatString=gain = %<gain>\noffset = %<offset>
  Gain : Gain  Gain=100  ParameterDataType=sfix(16)  ParameterScaling=2^0  OutDataType=sfix(16)  OutScaling=2^0  OutDataTypeStr=Inherit: Same as input  ParamDataTypeStr=Inherit: Same as input
  Gain2 : Gain  Gain=k_sync  ParameterDataType=sfix(16)  ParameterScaling=2^0  OutDataType=sfix(16)  OutScaling=2^0  OutDataTypeStr=Inherit: Same as input  ParamDataTypeStr=Inherit: Same as input
  Product : Product  Inputs=*/  OutDataType=sfix(16)  OutScaling=2^0  RndMeth=Simplest  OutDataTypeStr=Inherit: Same as first input
  Saturation : Saturate  UpperLimit=100  LowerLimit=-100
      settings: AttributesFormatString=max = %<UpperLimit>\nmin = %<LowerLimit>
  Saturation1 : Saturate  UpperLimit=100  LowerLimit=-100
      settings: AttributesFormatString=max = %<UpperLimit>\nmin = %<LowerLimit>
  Sum : Sum  Inputs=|++  OutDataType=sfix(16)  OutScaling=2^0  OutDataTypeStr=Inherit: Same as first input
  Sum1 : Sum  Inputs=|+-  OutDataType=sfix(16)  OutScaling=2^0  OutDataTypeStr=Inherit: Same as first input
  Sum2 : Sum  Inputs=|++  OutDataType=sfix(16)  OutScaling=2^0  OutDataTypeStr=Inherit: Same as first input
  Switch2 : Switch  Criteria=u2 ~= 0  OutDataType=sfix(16)  OutScaling=2^0
  Switch3 : Switch  Criteria=u2 ~= 0  OutDataType=sfix(16)  OutScaling=2^0
  pwm_l : Outport  OutDataType=sfix(16)  OutScaling=2^0
  pwm_r : Outport  Port=2  OutDataType=sfix(16)  OutScaling=2^0
  wires:
  Sum/1 -> Saturation/1
  pwm_turn/1 -> Sum/2, Sum1/2
  Gain/1 -> Friction Compensator/1
  Saturation1/1 -> pwm_r/1
  Saturation/1 -> pwm_l/1
  vol/1 -> Product/1
  Product/1 -> Gain/1
  Cal theta_diff/1(theta_diff) -> Gain2/1
  Switch3/1 -> Switch2/2, Cal theta_diff/1(flag_turn)
  Constant1/1 -> Switch2/1
  Gain2/1 -> Switch2/3
  battery/1 -> Cal vol_max/1(battery)
  Cal vol_max/1(vol_max) -> Product/2
  Sum1/1 -> Sum2/1
  Sum2/1 -> Saturation1/1
  Switch2/1 -> Sum2/2
  Friction Compensator/1 -> Sum1/1, Sum/1
  theta_m_l/1 -> Cal theta_diff/2(theta_m_l)
  theta_m_r/1 -> Cal theta_diff/3(theta_m_r)
  Constant5/1 -> Switch3/1
  Constant6/1 -> Switch3/3
  phidot_cmd/1 -> Data Type Conversion2/1
  Data Type Conversion2/1 -> Switch3/2

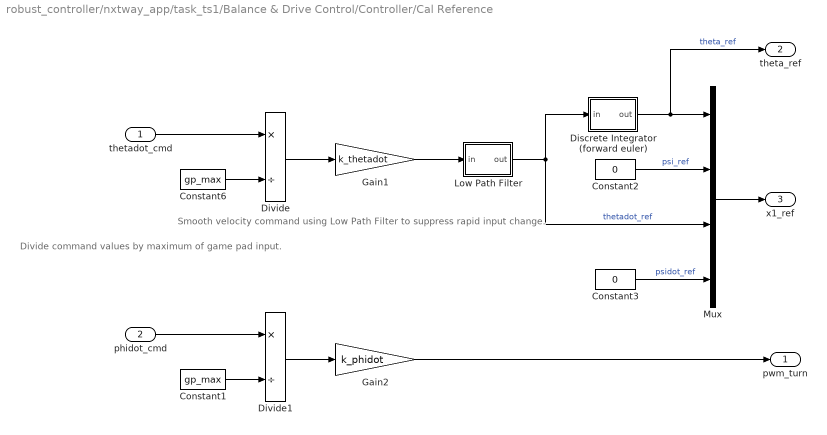
== system robust_controller/nxtway_app/task_ts1/Balance & Drive Control/Controller/Cal Reference ==
  note: Divide command values by
      | maximum of game pad input.
  note: Smooth velocity command
      | using Low Path Filter to
      | suppress rapid input change.
  thetadot_cmd : Inport
  phidot_cmd : Inport  Port=2
  Constant1 : Constant  Value=gp_max  VectorParams1D=off  OutDataTypeMode=int8  OutDataType=FIXDT  OutScaling=2^0  OutDataTypeStr=int8  SampleTime=-1
      settings: AttributesFormatString=DataType = %<OutDataTypeStr>
  Constant2 : Constant  Value=0  VectorParams1D=off  OutDataTypeMode=single  OutDataType=FIXDT  OutScaling=2^0  OutDataTypeStr=single  SampleTime=-1
      settings: AttributesFormatString=DataType = %<OutDataTypeStr>
  Constant3 : Constant  Value=0  VectorParams1D=off  OutDataTypeMode=single  OutDataType=FIXDT  OutScaling=2^0  OutDataTypeStr=single  SampleTime=-1
      settings: AttributesFormatString=DataType = %<OutDataTypeStr>
  Constant6 : Constant  Value=gp_max  VectorParams1D=off  OutDataTypeMode=int8  OutDataType=FIXDT  OutScaling=2^0  OutDataTypeStr=int8  SampleTime=-1
      settings: AttributesFormatString=DataType = %<OutDataTypeStr>
  Discrete Integrator (forward euler) : Subsystem
  Divide : Product  Inputs=*/  OutDataType=sfix(16)  OutScaling=2^-10  RndMeth=Simplest  OutDataTypeStr=Inherit: Same as first input
  Divide1 : Product  Inputs=*/  OutDataType=sfix(16)  OutScaling=2^-10  RndMeth=Simplest  OutDataTypeStr=Inherit: Same as first input
  Gain1 : Gain  Gain=k_thetadot  ParameterDataType=sfix(16)  ParameterScaling=2^0  OutDataType=sfix(16)  OutScaling=2^0  OutDataTypeStr=Inherit: Same as input  ParamDataTypeStr=Inherit: Same as input
  Gain2 : Gain  Gain=k_phidot  ParameterDataType=sfix(16)  ParameterScaling=2^0  OutDataType=sfix(16)  OutScaling=2^0  OutDataTypeStr=Inherit: Same as input  ParamDataTypeStr=Inherit: Same as input
  Low Path Filter : Subsystem
  Mux : Mux
  pwm_turn : Outport
  theta_ref : Outport  Port=2
  x1_ref : Outport  Port=3
  wires:
  phidot_cmd/1 -> Divide1/1
  Gain1/1 -> Low Path Filter/1(in)
  thetadot_cmd/1 -> Divide/1
  Divide/1 -> Gain1/1
  Gain2/1 -> pwm_turn/1
  Constant1/1 -> Divide1/2
  Divide1/1 -> Gain2/1
  Mux/1 -> x1_ref/1
  Discrete Integrator (forward euler)/1(out) -> theta_ref/1, Mux/1  "theta_ref"
  Constant2/1 -> Mux/2  "psi_ref"
  Constant3/1 -> Mux/4  "psidot_ref"
  Low Path Filter/1(out) -> Mux/3, Discrete Integrator (forward euler)/1(in)  "thetadot_ref"
  Constant6/1 -> Divide/2

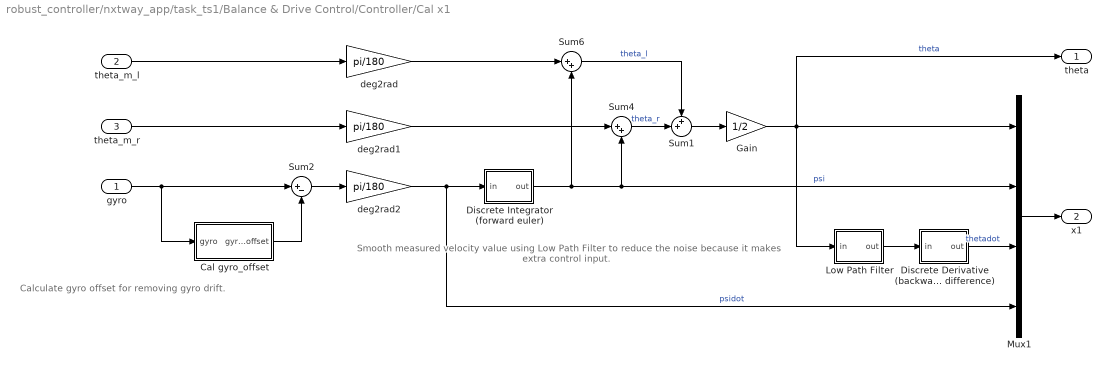
== system robust_controller/nxtway_app/task_ts1/Balance & Drive Control/Controller/Cal x1 ==
  note: Smooth measured velocity value using
      | Low Path Filter to reduce the noise
      | because it makes extra control input.
  note: Calculate gyro offset for removing gyro drift.
  gyro : Inport  OutDataType=sfix(16)  OutScaling=2^0
  theta_m_l : Inport  Port=2  OutDataType=sfix(16)  OutScaling=2^0
  theta_m_r : Inport  Port=3  OutDataType=sfix(16)  OutScaling=2^0
  Cal gyro_offset : Subsystem
  Discrete Derivative (backward difference) : Subsystem
  Discrete Integrator (forward euler) : Subsystem
  Gain : Gain  Gain=1/2  ParameterDataType=sfix(16)  ParameterScaling=2^0  OutDataType=sfix(16)  OutScaling=2^0  OutDataTypeStr=Inherit: Same as input  ParamDataTypeStr=Inherit: Same as input
  Low Path Filter : Subsystem
  Mux1 : Mux
  Sum1 : Sum  Inputs=++|  OutDataType=sfix(16)  OutScaling=2^0  OutDataTypeStr=Inherit: Same as first input
  Sum2 : Sum  Inputs=|+-  OutDataType=sfix(16)  OutScaling=2^0  OutDataTypeStr=Inherit: Same as first input
  Sum4 : Sum  Inputs=|++  OutDataType=sfix(16)  OutScaling=2^0  OutDataTypeStr=Inherit: Same as first input
  Sum6 : Sum  Inputs=|++  OutDataType=sfix(16)  OutScaling=2^0  OutDataTypeStr=Inherit: Same as first input
  deg2rad : Gain  Gain=pi/180  ParameterDataType=sfix(16)  ParameterScaling=2^0  OutDataType=sfix(16)  OutScaling=2^0  OutDataTypeStr=Inherit: Same as input  ParamDataTypeStr=Inherit: Same as input
  deg2rad1 : Gain  Gain=pi/180  ParameterDataType=sfix(16)  ParameterScaling=2^0  OutDataType=sfix(16)  OutScaling=2^0  OutDataTypeStr=Inherit: Same as input  ParamDataTypeStr=Inherit: Same as input
  deg2rad2 : Gain  Gain=pi/180  ParameterDataType=sfix(16)  ParameterScaling=2^0  OutDataType=sfix(16)  OutScaling=2^0  OutDataTypeStr=Inherit: Same as input  ParamDataTypeStr=Inherit: Same as input
  theta : Outport  OutDataType=sfix(16)  OutScaling=2^0
  x1 : Outport  Port=2  OutDataType=sfix(16)  OutScaling=2^0
  wires:
  deg2rad1/1 -> Sum4/1
  Mux1/1 -> x1/1
  Discrete Integrator (forward euler)/1(out) -> Sum6/2, Sum4/2, Mux1/2  "psi"
  deg2rad/1 -> Sum6/1
  theta_m_l/1 -> deg2rad/1
  theta_m_r/1 -> deg2rad1/1
  Discrete Derivative (backward difference)/1(out) -> Mux1/3  "thetadot"
  Sum6/1 -> Sum1/1  "theta_l"
  Sum4/1 -> Sum1/2  "theta_r"
  Sum1/1 -> Gain/1
  gyro/1 -> Sum2/1, Cal gyro_offset/1(gyro)
  Sum2/1 -> deg2rad2/1
  deg2rad2/1 -> Discrete Integrator (forward euler)/1(in), Mux1/4  "psidot"
  Low Path Filter/1(out) -> Discrete Derivative (backward difference)/1(in)
  Cal gyro_offset/1(gyro_offset) -> Sum2/2
  Gain/1 -> theta/1, Mux1/1, Low Path Filter/1(in)  "theta"

== system robust_controller/nxtway_app/task_ts1/Balance & Drive Control/Controller/Discrete Integrator (forward euler) ==
  in : Inport  OutDataType=sfix(16)  OutScaling=2^0
  Gain : Gain  Gain=ts1  ParameterDataType=sfix(16)  ParameterScaling=2^0  OutDataType=sfix(16)  OutScaling=2^0  OutDataTypeStr=Inherit: Same as input  ParamDataTypeStr=Inherit: Same as input
  Sum : Sum  Inputs=|++  OutDataType=sfix(16)  OutScaling=2^0  OutDataTypeStr=Inherit: Same as first input
  Unit Delay : UnitDelay  SampleTime=-1
  out : Outport  OutDataType=sfix(16)  OutScaling=2^0
  wires:
  in/1 -> Gain/1
  Sum/1 -> Unit Delay/1
  Gain/1 -> Sum/1
  Unit Delay/1 -> out/1, Sum/2

== system robust_controller/nxtway_app/task_ts1/Balance & Drive Control/Data Logging/Scaling ==
  note: LSB means scaling value.
      | You need to multiply log data by LSB to get phisical value.
  psi_single : Inport
  Divide : Product  Inputs=*/  OutDataType=sfix(16)  OutScaling=2^-10  RndMeth=Simplest  OutDataTypeStr=Inherit: Same as first input
  LSB : Constant  Value=2^-10  VectorParams1D=off  OutDataTypeMode=single  OutDataType=FIXDT  OutScaling=2^0  OutDataTypeStr=single  SampleTime=-1
      settings: AttributesFormatString=DataType = %<OutDataTypeStr>
  rad2deg : Gain  Gain=180/pi  ParameterDataType=sfix(16)  ParameterScaling=2^0  OutDataType=sfix(16)  OutScaling=2^0  OutDataTypeStr=Inherit: Same as input  ParamDataTypeStr=Inherit: Same as input
  psi_int : Outport
  wires:
  LSB/1 -> Divide/2
  rad2deg/1 -> Divide/1
  psi_single/1 -> rad2deg/1
  Divide/1 -> psi_int/1

== system robust_controller/nxtway_app/task_ts1/Balance & Drive Control/Make Command/Cal Command ==
  note: NXTway-GS rotates right when it is avoiding obstacle.
  flag_avoid : Inport
  Constant : Constant  Value=gp_max  VectorParams1D=off  OutDataTypeMode=int8  OutDataType=FIXDT  OutScaling=2^0  OutDataTypeStr=int8  SampleTime=-1
      settings: AttributesFormatString=DataType = %<OutDataTypeStr>
  Constant1 : Constant  Value=4*pi/180  VectorParams1D=off  OutDataTypeMode=int8  OutDataType=FIXDT  OutScaling=2^0  OutDataTypeStr=int8  SampleTime=-1
      settings: AttributesFormatString=DataType = %<OutDataTypeStr>
  Constant2 : Constant  Value=0  VectorParams1D=off  OutDataTypeMode=int8  OutDataType=FIXDT  OutScaling=2^0  OutDataTypeStr=int8  SampleTime=-1
      settings: AttributesFormatString=DataType = %<OutDataTypeStr>
  Constant3 : Constant  Value=gp_max  VectorParams1D=off  OutDataTypeMode=int8  OutDataType=FIXDT  OutScaling=2^0  OutDataTypeStr=int8  SampleTime=-1
      settings: AttributesFormatString=DataType = %<OutDataTypeStr>
  Switch : Switch  Criteria=u2 ~= 0  OutDataType=sfix(16)  OutScaling=2^0
  Switch2 : Switch  Criteria=u2 ~= 0  OutDataType=sfix(16)  OutScaling=2^0
  thetadot_cmd : Outport
  phidot_cmd : Outport  Port=2
  wires:
  flag_avoid/1 -> Switch2/2, Switch/2  "flag_turn"
  Constant1/1 -> Switch/1
  Constant/1 -> Switch/3
  Constant3/1 -> Switch2/1
  Constant2/1 -> Switch2/3
  Switch/1 -> thetadot_cmd/1
  Switch2/1 -> phidot_cmd/1

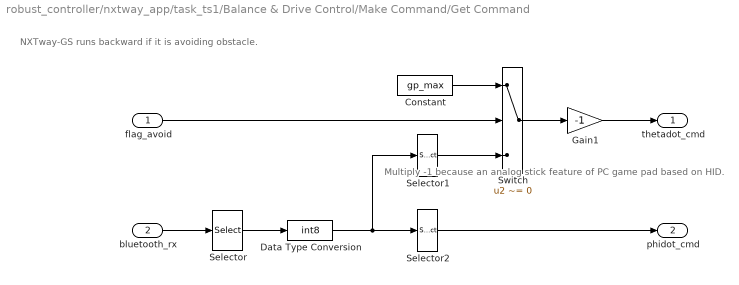
== system robust_controller/nxtway_app/task_ts1/Balance & Drive Control/Make Command/Get Command ==
  note: Multiply -1 because an analog stick
      | feature of PC game pad based on HID.
  note: NXTway-GS runs backward if it is avoiding obstacle.
  flag_avoid : Inport
  bluetooth_rx : Inport  Port=2
  Constant : Constant  Value=gp_max  VectorParams1D=off  OutDataTypeMode=int8  OutDataType=FIXDT  OutScaling=2^0  OutDataTypeStr=int8  SampleTime=-1
      settings: AttributesFormatString=DataType = %<OutDataTypeStr>
  Data Type Conversion : DataTypeConversion  OutDataTypeMode=int8  OutDataType=sfix(16)  OutScaling=2^0  OutDataTypeStr=int8  RndMeth=Simplest
      settings: AttributesFormatString=Round = %<RndMeth>
  Gain1 : Gain  Gain=-1  ParameterDataType=sfix(16)  ParameterScaling=2^0  OutDataType=sfix(16)  OutScaling=2^0  OutDataTypeStr=Inherit: Same as input  ParamDataTypeStr=Inherit: Same as input
  Selector : Selector  InputPortWidth=32  IndexOptions=Index vector (dialog)  Indices=[1 2]  OutputSizes=1
      settings: AttributesFormatString=Indices = %<Indices>
  Selector1 : Selector  InputPortWidth=2  IndexOptions=Index vector (dialog)  Indices=1  OutputSizes=1
  Selector2 : Selector  InputPortWidth=2  IndexOptions=Index vector (dialog)  Indices=2  OutputSizes=1
  Switch : Switch  Criteria=u2 ~= 0  OutDataType=sfix(16)  OutScaling=2^0
  thetadot_cmd : Outport
  phidot_cmd : Outport  Port=2
  wires:
  Selector/1 -> Data Type Conversion/1
  Data Type Conversion/1 -> Selector2/1, Selector1/1
  Selector1/1 -> Switch/3
  bluetooth_rx/1 -> Selector/1
  Selector2/1 -> phidot_cmd/1
  Switch/1 -> Gain1/1
  Constant/1 -> Switch/1
  Gain1/1 -> thetadot_cmd/1
  flag_avoid/1 -> Switch/2

== system robust_controller/nxtway_app/task_ts1/Balance & Drive Control/Controller/Cal PWM/Cal theta_diff ==
  note: Detect turn -> straight run change
  note: Save the difference between
      | left and right motor revolution angle
  flag_turn : Inport
  theta_m_l : Inport  Port=2
  theta_m_r : Inport  Port=3
  Detect Flag Falling : Subsystem
  Set theta_offset : Subsystem
  Sum1 : Sum  Inputs=|+-  OutDataType=sfix(16)  OutScaling=2^0  OutDataTypeStr=Inherit: Same as first input
  Sum5 : Sum  Inputs=|-+  OutDataType=sfix(16)  OutScaling=2^0  OutDataTypeStr=Inherit: Same as first input
  theta_diff : Outport
  wires:
  flag_turn/1 -> Detect Flag Falling/1(flag)
  Sum5/1 -> theta_diff/1
  Detect Flag Falling/1(falling) -> Set theta_offset/Enable
  Sum1/1 -> Set theta_offset/1(theta_diff), Sum5/2
  theta_m_l/1 -> Sum1/1
  theta_m_r/1 -> Sum1/2
  Set theta_offset/1(theta_offset) -> Sum5/1

== system robust_controller/nxtway_app/task_ts1/Balance & Drive Control/Controller/Cal PWM/Cal vol_max ==
  battery : Inport
  Constant : Constant  Value=0.625  OutDataTypeMode=single  OutDataType=sfix(16)  OutScaling=2^0  OutDataTypeStr=single  SampleTime=-1
      settings: AttributesFormatString=DataType = %<OutDataTypeStr>
  Gain3 : Gain  Gain=0.001089  ParameterDataType=sfix(16)  ParameterScaling=2^0  OutDataType=sfix(16)  OutScaling=2^0  OutDataTypeStr=Inherit: Same as input  ParamDataTypeStr=Inherit: Same as input
  Sum2 : Sum  Inputs=|+-  OutDataType=sfix(16)  OutScaling=2^0  OutDataTypeStr=Inherit: Same as first input
  vol_max : Outport
  wires:
  Constant/1 -> Sum2/2
  Sum2/1 -> vol_max/1
  Gain3/1 -> Sum2/1
  battery/1 -> Gain3/1

== system robust_controller/nxtway_app/task_ts1/Balance & Drive Control/Controller/Cal Reference/Discrete Integrator (forward euler) ==
  in : Inport  OutDataType=sfix(16)  OutScaling=2^0
  Gain : Gain  Gain=ts1  ParameterDataType=sfix(16)  ParameterScaling=2^0  OutDataType=sfix(16)  OutScaling=2^0  OutDataTypeStr=Inherit: Same as input  ParamDataTypeStr=Inherit: Same as input
  Sum : Sum  Inputs=|++  OutDataType=sfix(16)  OutScaling=2^0  OutDataTypeStr=Inherit: Same as first input
  Unit Delay : UnitDelay  SampleTime=-1
  out : Outport  OutDataType=sfix(16)  OutScaling=2^0
  wires:
  Unit Delay/1 -> Sum/2, out/1
  Gain/1 -> Sum/1
  Sum/1 -> Unit Delay/1
  in/1 -> Gain/1
